simulink model "sg_ClosedLoop_PID_float"  (Simulink 7.8)
settings: Solver=FixedStepDiscrete  SolverMode=SingleTasking  StartTime=0.0  StopTime=N*II  RelTol=1e-3
StopFcn:
  | sg_ClosedLoop_PID_float_StopFcn
undefined symbols (not defined in the file or in its folder): C, Gd, Gi, Gp, II, max_clip, min_clip
libraries: xbsIndex_r4 x41
settings Model: Creator=danieleb  LastModifiedBy=danieleb
settings DebuggingCC: AlgebraicLoopMsg=none

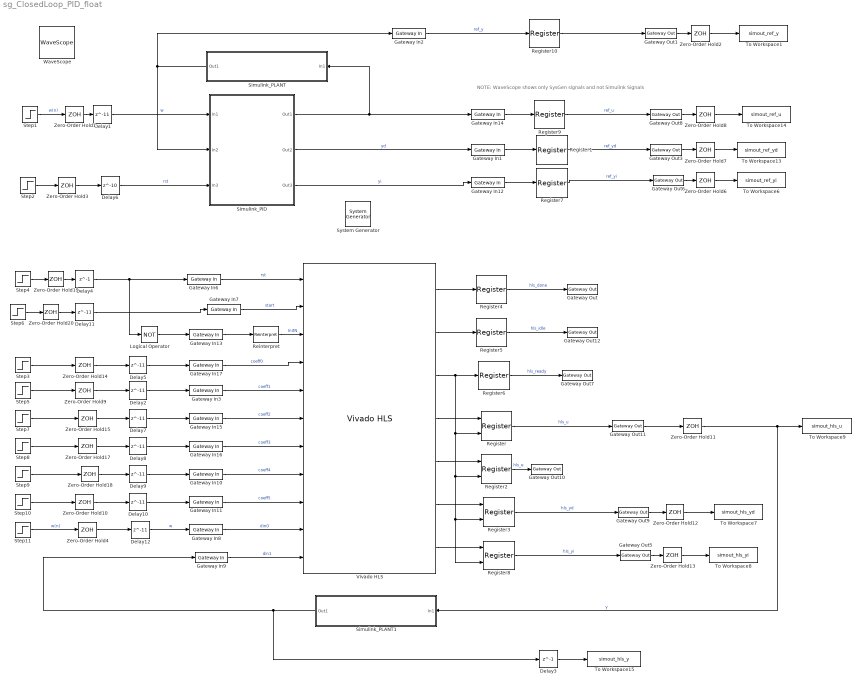
== system sg_ClosedLoop_PID_float ==
  note: NOTE: WaveScope shows only SysGen signals and not Simulink Signals
  " System Generator" : xbsIndex_r4/ System Generator  Tag=genX  xilinxfamily=zynq  part=xc7z020  speed=-1  package=clg400  synthesis_tool=XST  clock_wrapper=Clock Enables  directory=./netlist_top_PID  proj_type=Project Navigator  Synth_file=XST Defaults  Impl_file=ISE Defaults  testbench=off  simulink_period=1  sysclk_period=10  dcm_input_clock_period=10  incr_netlist=off  trim_vbits=Everywhere in SubSystem  dbl_ovrd=According to Block Masks  core_generation=According to Block Masks  run_coregen=off  deprecated_control=off  eval_field=0  block_type=sysgen
  Delay{1..2,5,7..12} (9 alike) : Delay  DelayLength=11
  Delay3 : Delay  DelayLength=1
  Delay4 : Delay  DelayLength=1
  Delay6 : Delay  DelayLength=10
  Gateway In{1..3,8..12,14..17} (12 alike) : xbsIndex_r4/Gateway In  gui_display_data_type=Floating-point  arith_type=Floating-point  n_bits=25  bin_pt=25-10  preci_type=Single  exp_width=8  frac_width=24  quantization="Round  (unbiased: +/- Inf)"  overflow=Saturate  period=II  dbl_ovrd=off  timing_constraint=None  locs_specified=off  LOCs={}  UseAsADC=off  ADCChannel='1'  inherit_from_input=off  hdl_port=on  block_type=gatewayin
  Gateway In13 : xbsIndex_r4/Gateway In  gui_display_data_type=Boolean  arith_type=Boolean  n_bits=25  bin_pt=25-10  preci_type=Single  exp_width=8  frac_width=24  quantization="Round  (unbiased: +/- Inf)"  overflow=Saturate  period=II  dbl_ovrd=off  timing_constraint=None  locs_specified=off  LOCs={}  UseAsADC=off  ADCChannel='1'  inherit_from_input=off  hdl_port=on  block_type=gatewayin
  Gateway In6 : xbsIndex_r4/Gateway In  gui_display_data_type=Boolean  arith_type=Boolean  n_bits=25  bin_pt=25-10  preci_type=Single  exp_width=8  frac_width=24  quantization="Round  (unbiased: +/- Inf)"  overflow=Saturate  period=II  dbl_ovrd=off  timing_constraint=None  locs_specified=off  LOCs={}  UseAsADC=off  ADCChannel='1'  inherit_from_input=off  hdl_port=on  block_type=gatewayin
  Gateway In7 : xbsIndex_r4/Gateway In  gui_display_data_type=Boolean  arith_type=Boolean  n_bits=25  bin_pt=25-10  preci_type=Single  exp_width=8  frac_width=24  quantization="Round  (unbiased: +/- Inf)"  overflow=Saturate  period=II  dbl_ovrd=off  timing_constraint=None  locs_specified=off  LOCs={}  UseAsADC=off  ADCChannel='1'  inherit_from_input=off  hdl_port=on  block_type=gatewayin
  Gateway Out{,1,3,5..6,8..10,12} (9 alike) : xbsIndex_r4/Gateway Out  inherit_from_input=off  hdl_port=off  timing_constraint=None  locs_specified=off  LOCs={}  UseAsDAC=off  DACChannel='1'  block_type=gatewayout
  Gateway Out11 : xbsIndex_r4/Gateway Out  inherit_from_input=off  hdl_port=on  timing_constraint=None  locs_specified=off  LOCs={}  UseAsDAC=off  DACChannel='1'  block_type=gatewayout
  Gateway Out7 : xbsIndex_r4/Gateway Out  inherit_from_input=off  hdl_port=on  timing_constraint=None  locs_specified=off  LOCs={}  UseAsDAC=off  DACChannel='1'  block_type=gatewayout
  Logical Operator : Logic  Operator=NOT  AllPortsSameDT=off  OutDataTypeStr=boolean
  Register{,2..3,8} (4 alike) : xbsIndex_r4/Register  init=0  rst=off  en=on  dbl_ovrd=off  block_type=register
  Register{1,4..7,9..10} (7 alike) : xbsIndex_r4/Register  init=0  rst=off  en=off  dbl_ovrd=off  block_type=register
  Reinterpret : xbsIndex_r4/Reinterpret  force_arith_type=on  arith_type=Unsigned  force_bin_pt=on  bin_pt=0  block_type=reinterpret
  Simulink_PID : Subsystem
  Simulink_PLANT : Subsystem
  Simulink_PLANT1 : Subsystem
  Step1 : Step  After=10  SampleTime=II
  Step10 : Step  After=min_clip  SampleTime=II
  Step11 : Step  After=10  SampleTime=II
  Step2 : Step  Before=1  After=0  SampleTime=II
  Step3 : Step  After=Gi  SampleTime=II
  Step4 : Step  Before=1  After=0  SampleTime=II
  Step5 : Step  After=Gd  SampleTime=II
  Step6 : Step  SampleTime=II
  Step7 : Step  After=C  SampleTime=II
  Step8 : Step  After=Gp  SampleTime=II
  Step9 : Step  After=max_clip  SampleTime=II
  To Workspace1 : ToWorkspace  VariableName=simout_ref_y  SampleTime=-1  SaveFormat=Array
  To Workspace13 : ToWorkspace  VariableName=simout_ref_yd  SampleTime=-1  SaveFormat=Array
  To Workspace14 : ToWorkspace  VariableName=simout_ref_u  SampleTime=-1  SaveFormat=Array
  To Workspace15 : ToWorkspace  VariableName=simout_hls_y  SampleTime=-1  SaveFormat=Array
  To Workspace6 : ToWorkspace  VariableName=simout_ref_yi  SampleTime=-1  SaveFormat=Array
  To Workspace7 : ToWorkspace  VariableName=simout_hls_yd  SampleTime=-1  SaveFormat=Array
  To Workspace8 : ToWorkspace  VariableName=simout_hls_yi  SampleTime=-1  SaveFormat=Array
  To Workspace9 : ToWorkspace  VariableName=simout_hls_u  SampleTime=-1  SaveFormat=Array
  Vivado HLS : xbsIndex_r4/Vivado HLS  anytable='C:/BagniD/work/xapp_pid/hls/floatp/hls_floatp_pid_prj/solution3_test/'  display_datatype=off  rate_propagation_method=Simulink system period  model_file_path=''  latency=1  block_type=hls
      settings: infoedit=This block allows including C,C++ and SystemC source files in System Generator for DSP designs.
  WaveScope : xbsIndex_r4/WaveScope  block_type=wavescope
  Zero-Order Hold{1..4,6..8,11..13,19..20} (12 alike) : ZeroOrderHold  SampleTime=II
  Zero-Order Hold{9..10,14..15,17..18} (6 alike) : ZeroOrderHold  SampleTime=-1
  wires:
  Simulink_PID/1(Out1) -> Gateway In14/1, Simulink_PLANT/1(In1)
  Simulink_PID/2(Out2) -> Gateway In1/1  "yd"
  Step1/1 -> Zero-Order Hold1/1  "w(n)"
  Delay1/1 -> Simulink_PID/1(In1)  "w"
  Zero-Order Hold1/1 -> Delay1/1
  Simulink_PID/3(Out3) -> Gateway In12/1  "yi"
  Step2/1 -> Zero-Order Hold3/1
  Zero-Order Hold3/1 -> Delay6/1
  Delay6/1 -> Simulink_PID/3(In3)  "rst"
  Gateway In6/1 -> Vivado HLS/1  "rst"
  Delay4/1 -> Gateway In6/1, Logical Operator/1
  Delay11/1 -> Gateway In7/1
  Delay5/1 -> Gateway In17/1
  Gateway In17/1 -> Vivado HLS/4  "coeff0"
  Gateway In7/1 -> Vivado HLS/2  "start"
  Reinterpret/1 -> Vivado HLS/3  "InitN"
  Zero-Order Hold14/1 -> Delay5/1
  Step3/1 -> Zero-Order Hold14/1
  Delay2/1 -> Gateway In3/1
  Gateway In3/1 -> Vivado HLS/5  "coeff1"
  Zero-Order Hold9/1 -> Delay2/1
  Step5/1 -> Zero-Order Hold9/1
  Gateway In8/1 -> Vivado HLS/10  "din0"
  Gateway In9/1 -> Vivado HLS/11  "din1"
  Gateway In13/1 -> Reinterpret/1
  Logical Operator/1 -> Gateway In13/1
  Gateway In15/1 -> Vivado HLS/6  "coeff2"
  Gateway In16/1 -> Vivado HLS/7  "coeff3"
  Gateway In10/1 -> Vivado HLS/8  "coeff4"
  Gateway In11/1 -> Vivado HLS/9  "coeff5"
  Delay7/1 -> Gateway In15/1
  Delay8/1 -> Gateway In16/1
  Delay9/1 -> Gateway In10/1
  Delay10/1 -> Gateway In11/1
  Zero-Order Hold15/1 -> Delay7/1
  Zero-Order Hold17/1 -> Delay8/1
  Step7/1 -> Zero-Order Hold15/1
  Step8/1 -> Zero-Order Hold17/1
  Zero-Order Hold18/1 -> Delay9/1
  Step9/1 -> Zero-Order Hold18/1
  Zero-Order Hold10/1 -> Delay10/1
  Step10/1 -> Zero-Order Hold10/1
  Register/1 -> Gateway Out11/1  "hls_u"
  Register2/1 -> Gateway Out10/1  "hls_e"
  Register3/1 -> Gateway Out9/1  "hls_yd"
  Register4/1 -> Gateway Out/1  "hls_done"
  Register5/1 -> Gateway Out12/1  "hls_idle"
  Register6/1 -> Gateway Out7/1  "hls_ready"
  Register8/1 -> Gateway Out5/1  "hls_yi"
  Gateway Out9/1 -> Zero-Order Hold12/1
  Gateway Out5/1 -> Zero-Order Hold13/1
  Gateway Out11/1 -> Zero-Order Hold11/1
  Vivado HLS/1 -> Register4/1
  Vivado HLS/2 -> Register5/1
  Vivado HLS/3 -> Register6/1, Register/2, Register2/2, Register3/2, Register8/2
  Vivado HLS/4 -> Register/1
  Vivado HLS/5 -> Register2/1
  Vivado HLS/6 -> Register3/1
  Vivado HLS/7 -> Register8/1
  Zero-Order Hold11/1 -> To Workspace9/1, Simulink_PLANT1/1(In1)  "y"
  Zero-Order Hold12/1 -> To Workspace7/1
  Zero-Order Hold13/1 -> To Workspace8/1
  Step4/1 -> Zero-Order Hold19/1
  Zero-Order Hold19/1 -> Delay4/1
  Step6/1 -> Zero-Order Hold20/1
  Zero-Order Hold20/1 -> Delay11/1
  Step11/1 -> Zero-Order Hold4/1  "w(n)"
  Delay12/1 -> Gateway In8/1  "w"
  Zero-Order Hold4/1 -> Delay12/1
  Register7/1 -> Gateway Out6/1  "ref_yi"
  Gateway In12/1 -> Register7/1
  Gateway Out6/1 -> Zero-Order Hold6/1
  Gateway Out8/1 -> Zero-Order Hold8/1
  Gateway In14/1 -> Register9/1
  Register9/1 -> Gateway Out8/1  "ref_u"
  Register1/1 -> Gateway Out3/1  "ref_yd"
  Gateway Out3/1 -> Zero-Order Hold7/1
  Gateway In1/1 -> Register1/1
  Zero-Order Hold6/1 -> To Workspace6/1
  Zero-Order Hold7/1 -> To Workspace13/1
  Zero-Order Hold8/1 -> To Workspace14/1
  Simulink_PLANT1/1(Out1) -> Gateway In9/1, Delay3/1
  Simulink_PLANT/1(Out1) -> Simulink_PID/2(In2), Gateway In2/1
  Gateway Out1/1 -> Zero-Order Hold2/1
  Gateway In2/1 -> Register10/1  "ref_y"
  Register10/1 -> Gateway Out1/1
  Zero-Order Hold2/1 -> To Workspace1/1
  Delay3/1 -> To Workspace15/1

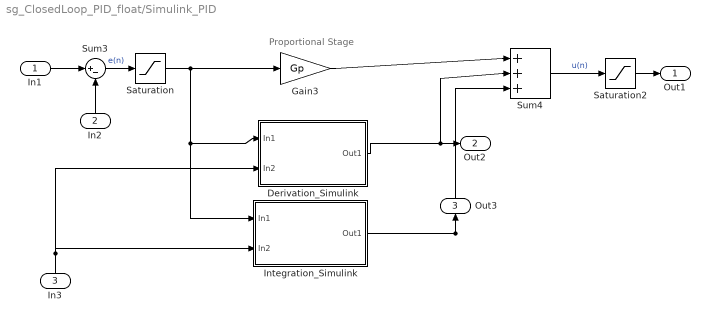
== system sg_ClosedLoop_PID_float/Simulink_PID ==
  note: Proportional Stage
  In1 : Inport
  In2 : Inport  Port=2
  In3 : Inport  Port=3
  Derivation_Simulink : Subsystem
  Gain3 : Gain  Gain=Gp
  Integration_Simulink : Subsystem
  Saturation : Saturate  UpperLimit=max_clip  LowerLimit=min_clip
  Saturation2 : Saturate  UpperLimit=max_clip  LowerLimit=min_clip
  Sum3 : Sum  Inputs=|+-
  Sum4 : Sum  Inputs=|+++
  Out1 : Outport
  Out2 : Outport  Port=2
  Out3 : Outport  Port=3
  wires:
  Gain3/1 -> Sum4/1
  Sum3/1 -> Saturation/1  "e(n)"
  Sum4/1 -> Saturation2/1  "u(n)"
  Saturation/1 -> Gain3/1, Derivation_Simulink/1(In1), Integration_Simulink/1(In1)
  Derivation_Simulink/1(Out1) -> Sum4/2, Out2/1
  Integration_Simulink/1(Out1) -> Sum4/3, Out3/1
  In1/1 -> Sum3/1
  In2/1 -> Sum3/2
  In3/1 -> Integration_Simulink/2(In2), Derivation_Simulink/2(In2)
  Saturation2/1 -> Out1/1

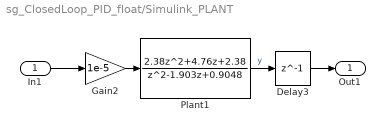
== system sg_ClosedLoop_PID_float/Simulink_PLANT ==
  In1 : Inport
  Delay3 : Delay  DelayLength=1
  Gain2 : Gain  Gain=1e-5
  Plant1 : DiscreteTransferFcn  Numerator=[2.38 4.76 2.38]  Denominator=[1 -1.903 0.9048]  SampleTime=II
  Out1 : Outport
  wires:
  Gain2/1 -> Plant1/1
  Plant1/1 -> Delay3/1  "y"
  In1/1 -> Gain2/1
  Delay3/1 -> Out1/1

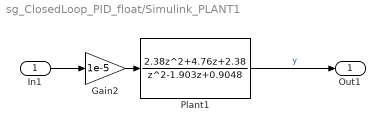
== system sg_ClosedLoop_PID_float/Simulink_PLANT1 ==
  In1 : Inport
  Gain2 : Gain  Gain=1e-5
  Plant1 : DiscreteTransferFcn  Numerator=[2.38 4.76 2.38]  Denominator=[1 -1.903 0.9048]  SampleTime=II
  Out1 : Outport
  wires:
  In1/1 -> Gain2/1
  Plant1/1 -> Out1/1  "y"
  Gain2/1 -> Plant1/1

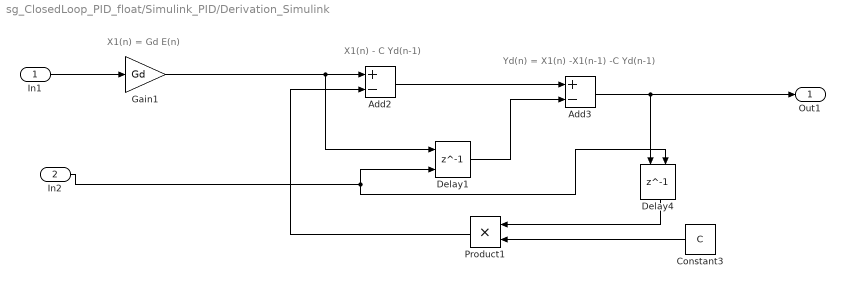
== system sg_ClosedLoop_PID_float/Simulink_PID/Derivation_Simulink ==
  note: X1(n) - C Yd(n-1)
  note: Yd(n) = X1(n) -X1(n-1) -C Yd(n-1)
  note: X1(n) = Gd E(n)
  In1 : Inport
  In2 : Inport  Port=2
  Add2 : Sum  Inputs=+-
  Add3 : Sum  Inputs=+-
  Constant3 : Constant  Value=C  OutDataTypeStr=single  SampleTime=II
  Delay1 : Delay  DelayLength=1  ExternalReset=Level hold
      settings: InputPortMap=u0,r5
  Delay4 : Delay  DelayLength=1  ExternalReset=Level hold
      settings: InputPortMap=u0,r5
  Gain1 : Gain  Gain=Gd
  Product1 : Product  RndMeth=Zero
  Out1 : Outport
  wires:
  In1/1 -> Gain1/1
  Delay1/1 -> Add3/2
  Add2/1 -> Add3/1
  Add3/1 -> Delay4/1, Out1/1
  Constant3/1 -> Product1/2
  Product1/1 -> Add2/2
  Delay4/1 -> Product1/1
  In2/1 -> Delay1/2, Delay4/2
  Gain1/1 -> Add2/1, Delay1/1

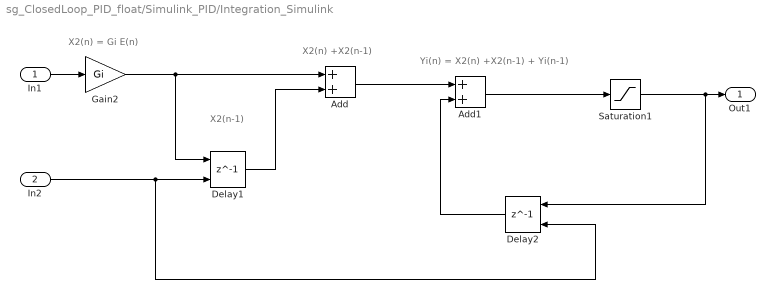
== system sg_ClosedLoop_PID_float/Simulink_PID/Integration_Simulink ==
  note: X2(n) = Gi E(n)
  note: X2(n) +X2(n-1)
  note: X2(n-1)
  note: Yi(n) = X2(n) +X2(n-1) + Yi(n-1)
  In1 : Inport
  In2 : Inport  Port=2
  Add : Sum
  Add1 : Sum
  Delay1 : Delay  DelayLength=1  ExternalReset=Level hold
      settings: InputPortMap=u0,r5
  Delay2 : Delay  DelayLength=1  ExternalReset=Level hold
      settings: InputPortMap=u0,r5
  Gain2 : Gain  Gain=Gi
  Saturation1 : Saturate  UpperLimit=max_clip  LowerLimit=min_clip
  Out1 : Outport
  wires:
  Add/1 -> Add1/1
  Add1/1 -> Saturation1/1
  Gain2/1 -> Add/1, Delay1/1
  Delay1/1 -> Add/2
  Saturation1/1 -> Out1/1, Delay2/1
  In1/1 -> Gain2/1
  Delay2/1 -> Add1/2
  In2/1 -> Delay1/2, Delay2/2
